simulink model "vehicle_animation_sim"  (R2017b)
settings: Solver=FixedStepAuto  StartTime=0  StopTime=45  FixedStep=0.01  RelTol=1e-3
values from neighbouring files (symbols this model uses):
  animation_update_interval = C*h_fixed    [setup.m]
  enable_CG_trace = 1    [setup.m]
  enable_rearAxle_trace = 1    [setup.m]
  plotAxisLimitMode = 0    [setup.m]
  plotAxisLimits = [-3 5 -3 6]*3    [setup.m]
  save_anim_frames = 0    [setup.m]
  vehicle_length = 1.64    [setup.m]
  vehicle_width = 0.86    [setup.m]
undefined symbols (not defined in the file or in its folder): datetime
libraries: simulink x1
settings Model: SimulationMode=rapid-accelerator  Creator=comperem  LastModifiedBy=cuc2a
settings DataIOCC: LimitDataPoints=on  SaveFormat=Array
settings OptimizationCC: BlockReduction=off  BooleanDataType=off  LifeSpan=inf
settings DebuggingCC: SaveWithParameterizedLinksMsg=none  UnderspecifiedInitializationDetection=Classic  MergeDetectMultiDrivingBlocksExec=none  SignalResolutionControl=TryResolveAllWithWarning  AllowSymbolicDim=off  SFUnexpectedBacktrackingDiag=warning  SFNoUnconditionalDefaultTransitionDiag=warning  SFExecutionAtInitializationDiag=none
settings HardwareCC: ProdBitPerPointer=32  ProdBitPerSizeT=32  ProdBitPerPtrDiffT=32  ProdLargestAtomicFloat=None  ProdIntDivRoundTo=Undefined  ProdEndianess=Unspecified  ProdWordSize=32  ProdHWDeviceType=32-bit Generic  TargetBitPerPointer=64  TargetBitPerSizeT=64  TargetBitPerPtrDiffT=64  TargetLongLongMode=on  TargetIntDivRoundTo=Zero  TargetEndianess=LittleEndian  TargetWordSize=64  TargetHWDeviceType=MATLAB Host  ProdEqTarget=off
settings ModelReferenceCC: PropagateSignalLabelsOutOfModel=off
settings CodeAppCC: StateflowObjectComments=on
settings GRTTargetCC: TargetLangStandard=C89/C90 (ANSI)  GeneratePreprocessorConditionals=Disable all
settings ConfigComp: CovMetricSettings=dw  CovHtmlReporting=on  CovSaveCumulativeToWorkspaceVar=on  CovSaveSingleToWorkspaceVar=on  CovExternalEMLEnable=off  CovSFcnEnable=off

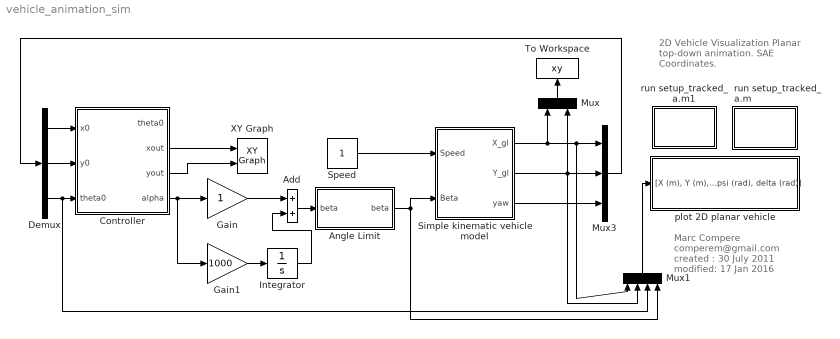
== system vehicle_animation_sim ==
  note: Marc Compere
      | comperem@gmail.com
      | created : 30 July 2011
      | modified: 17 Jan 2016
  note: 2D Vehicle Visualization
      | Planar top-down animation.
      | SAE Coordinates.
  Add : Sum
  Angle Limit : MATLAB Function  TreatAsAtomicUnit=on
  Controller : MATLAB Function  TreatAsAtomicUnit=on
  Demux : Demux  Outputs=3
  Gain : Gain
  Gain1 : Gain  Gain=1000
  Integrator : Integrator
  Mux : Mux  Inputs=2
  Mux1 : Mux
  Mux3 : Mux  Inputs=3
  "Simple kinematic vehicle model " : Subsystem
  Speed : Constant
  To Workspace : ToWorkspace  VariableName=xy  SampleTime=-1
      settings: Save2DSignal=2-D array (concatenate along first dimension)
  XY Graph : simulink/Sinks/XY Graph  xmin=-30  xmax=30  ymin=-30  ymax=30  st=-1
  plot 2D planar vehicle : Subsystem  mask(6DoF Animation){axisMode=plotAxisLimitMode, ax=plotAxisLimits, Ts=animation_update_interval, enable_CG_trace=enable_CG_trace, enable_rearAxle_trace=enable_rearAxle_trace, save_anim_frames=save_anim_frames, anim_frame_name_str=char(datetime('now','Format','yyyy-MM-dd_HH_mm_ss')), L=vehicle_length, W=vehicle_width}
      mask prompts: axisMode "Axis Mode (0->auto, 1->fixed, BOTH use Axes Limits below)"; ax "Axes limits [xmin xmax ymin ymax] (m):"; Ts "Time interval between updates (s):"; enable_CG_trace "Enable vehicle CG trace? (0/1)"; enable_rearAxle_trace "Enable rear axle trace? (0/1)"; save_anim_frames "Save animaton frames? (0/1)"; anim_frame_name_str "Animation sequence name (if save frames==1)"; L "Vehicle length (m)"; W "Vehicle width (m)"
      mask help:
      | Create a 2D animated view of a steering vehicle model with tires.
      |
      | Marc Compere
      | CompereM@saic.com
      | created : 22 August 2002
      | modified: 28 Dec 2015
      mask init:
      | Config.axisMode=axisMode;
      | Config.ax=ax;
      | Config.Ts=Ts;
      | Config.enable_CG_trace=enable_CG_trace;
      | Config.enable_rearAxle_trace=enable_rearAxle_trace;
      | Config.save_anim_frames=save_anim_frames;
      | Config.anim_frame_name_str=anim_frame_name_str;
      | Config.L=L;
      | Config.W=W;
      mask Help:
      | <p>This block generates a 3 dimensional display of a simulation trajectory, with the craft orientation displayed during flight</p>
      | 
      | <p>There are two inputs to this block, Position and Euler.  These inputs contain more than one signal as described below.</p>
      | 
      | <p><H4>Block Vector Input - Position</H4>
      | <ul>
      | <li>X Position</li>
      | <li>Y Position</li>
      | <li>Z Position</li>
      | </ul>
      | </p>
      | 
      | <p><H4>Block Vector Input - Euler</H4>
      |     <ul>
      |     <li>Roll Attitude</li>
      |     <li>Pitch Attitude</li>
      |     <li>Yaw Attitude</li>
      |    </ul>
      |    </p>
  run setup_tracked_a.m : Subsystem
      settings: OpenFcn=setup
      mask Display: fprintf('run setup.m')
  run setup_tracked_a.m1 : Subsystem
      settings: OpenFcn=edit setup
      mask Display: fprintf('edit setup.m')
  wires:
  "Simple kinematic vehicle model "/1(X_gl) -> Mux/1, Mux1/1, Mux3/1
  "Simple kinematic vehicle model "/2(Y_gl) -> Mux/2, Mux3/2, Mux1/2
  "Simple kinematic vehicle model "/3(yaw) -> Mux3/3
  Demux/1 -> Controller/1(x0)
  Demux/2 -> Controller/2(y0)
  Speed/1 -> "Simple kinematic vehicle model "/1(Speed)
  Gain/1 -> Add/1
  Angle Limit/1(beta) -> "Simple kinematic vehicle model "/2(Beta), Mux1/4
  Mux3/1 -> Demux/1
  Controller/2(xout) -> XY Graph/1
  Controller/3(yout) -> XY Graph/2
  Mux/1 -> To Workspace/1
  Controller/4(alpha) -> Gain1/1, Gain/1
  Mux1/1 -> plot 2D planar vehicle/1("[X (m), Y (m), psi (rad), delta (rad)]")
  Demux/3 -> Mux1/3, Controller/3("theta0 ")
  Gain1/1 -> Integrator/1
  Integrator/1 -> Add/2
  Add/1 -> Angle Limit/1("beta ")

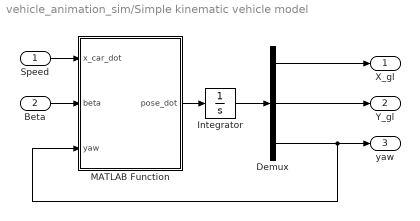
== system vehicle_animation_sim/Simple kinematic vehicle model  ==
  Speed : Inport
  Beta : Inport  Port=2
  Demux : Demux  Outputs=3
  Integrator : Integrator
  MATLAB Function : MATLAB Function  TreatAsAtomicUnit=on
  X_gl : Outport
  Y_gl : Outport  Port=2
  yaw : Outport  Port=3
  wires:
  Demux/1 -> X_gl/1
  Demux/3 -> MATLAB Function/3(yaw), yaw/1
  Demux/2 -> Y_gl/1
  Integrator/1 -> Demux/1
  MATLAB Function/1(pose_dot) -> Integrator/1
  Speed/1 -> MATLAB Function/1(x_car_dot)
  Beta/1 -> MATLAB Function/2(beta)

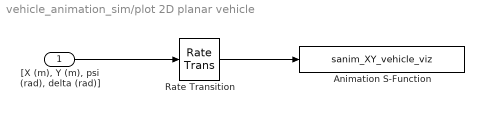
== system vehicle_animation_sim/plot 2D planar vehicle ==
  "[X (m), Y (m), psi (rad), delta (rad)]" : Inport
  Animation S-Function : S-Function  FunctionName=sanim_XY_vehicle_viz  Parameters=Config  SFunctionDeploymentMode=off  EnableBusSupport=off
  Rate Transition : RateTransition  Integrity=off
  wires:
  "[X (m), Y (m), psi (rad), delta (rad)]"/1 -> Rate Transition/1
  Rate Transition/1 -> Animation S-Function/1

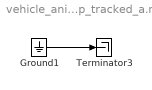
== system vehicle_animation_sim/run setup_tracked_a.m ==
  Ground1 : Ground
  Terminator3 : Terminator
  wires:
  Ground1/1 -> Terminator3/1

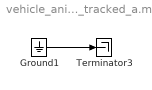
== system vehicle_animation_sim/run setup_tracked_a.m1 ==
  Ground1 : Ground
  Terminator3 : Terminator
  wires:
  Ground1/1 -> Terminator3/1

== matlab function vehicle_animation_sim/Controller ==
  data: theta0 output; xout output; x0 input; y0 input; theta0 input; yout output; PointMatrix parameter; alpha output
function [theta0,xout,yout,alpha] = fcn(x0,y0,theta0,PointMatrix)

% Define constants
LOWERDIST = 3.2;
UPPERDIST = 3.6;
VIEWING_ANGLE = 90*pi()/180;  %90 degrees in radians
WHEEL_BASE = 1.62;

% find the path length
szpm = size(PointMatrix);

% initialize the variables. 
xout = PointMatrix(szpm(1,1),1);
yout = PointMatrix(szpm(1,1),2);
alpha = 0;


for i = 1:szpm(1,1)
    %translate to the front of the cart.
    car_x = x0 + cos(theta0) * WHEEL_BASE;
    car_y = y0 + sin(theta0) * WHEEL_BASE;
    
    distance = sqrt((PointMatrix(i,1)-car_x)^2+(PointMatrix(i,2)-car_y)^2);

    if distance >= LOWERDIST && distance <= UPPERDIST 
        % creates a vector from the car front point to the pathpoint
        % substract our glabal position and the translation to the front. 
        pointVec = [PointMatrix(i,1)-x0-cos(theta0)*WHEEL_BASE ; PointMatrix(i,2)-y0-sin(theta0)*WHEEL_BASE];
        % creates a vector along the car
        carVec = [cos(theta0); sin(theta0)];
        
        % find the angle using the formular for finding angle between two
        % vectors.
        alpha = acos(dot(carVec,pointVec)/(norm(carVec)*norm(pointVec)));

        if alpha <= VIEWING_ANGLE/2
            xout = PointMatrix(i,1);
            yout = PointMatrix(i,2);
            %find the direction of the angle using the cross product.
            alpha = alpha * sign(carVec(1,1)*pointVec(2,1)-carVec(2,1)*pointVec(1,1));
            break %break the loop as soon as we find a point 
        end          
    end     
end

== matlab function vehicle_animation_sim/Simple kinematic vehicle model /MATLAB Function ==
  data: x_car_dot input; pose_dot output; beta input; yaw input
function pose_dot  = fcn(x_car_dot,beta,yaw)
W = 1.64;
theta = tan(beta)/W;
pose_dot = [cos(yaw)*x_car_dot
            sin(yaw)*x_car_dot
               theta*x_car_dot];

== matlab function vehicle_animation_sim/Angle Limit ==
  data: beta input; beta output
function beta = fcn(beta)

if beta > 22000/43408.5889
    beta = 22000/43408.5889;
    
elseif beta < -22000/43408.5889
    beta = -22000/43408.5889;  

end
